simulink model "AnotherOopsies"  (R2020a)
settings: Solver=FixedStepAuto  StartTime=0.0  StopTime=10.0  FixedStep=1e-3  RelTol=1e-3  EnableMultiTasking=on
undefined symbols (not defined in the file or in its folder): A0, A1, D0, D1, D10, D11, D12, D13, D2, D3, D4, D5, D6, D7, D8, D9, PTA0, PTA1, PTA2, PTB2, PTB23, PTB3, PTB9, PTC16, PTC17, PTC2, PTC3, PTC4, PTD0, PTD1, PTD2, PTD3
libraries: frdmk64flib x19, etargetslib x8, dspstat3 x1
settings Model: ExtModeTrigDuration=5  Creator=haque  LastModifiedBy=haque
settings OptimizationCC: EnhancedBackFolding=on  PassReuseOutputArgsAs=Individual arguments  ZeroExternalMemoryAtStartup=off  ZeroInternalMemoryAtStartup=off  MaxStackSize=64  OptimizeBlockOrder=speed  DifferentSizesBufferReuse=on  OptimizationCustomize=off  EfficientTunableParamExpr=on
settings DebuggingCC: ParameterTunabilityLossMsg=error
settings HardwareCC: ProdBitPerPointer=32  ProdBitPerSizeT=32  ProdBitPerPtrDiffT=32  ProdLargestAtomicInteger=Long  ProdLargestAtomicFloat=Double  ProdWordSize=32  ProdHWDeviceType=ARM Compatible->ARM Cortex
settings SFSimCC: MATLABDynamicMemAlloc=off
settings RTWCC: SystemTargetFile=ert.tlc  HardwareBoard=NXP FRDM-K64F  TemplateMakefile=ert_default_tmf  Toolchain=GNU Tools for ARM Embedded Processors
settings CodeAppCC: ForceParamTrailComments=on  IgnoreCustomStorageClasses=off  OperatorAnnotations=on  SimulinkDataObjDesc=on  SFDataObjDesc=on  InsertBlockDesc=on

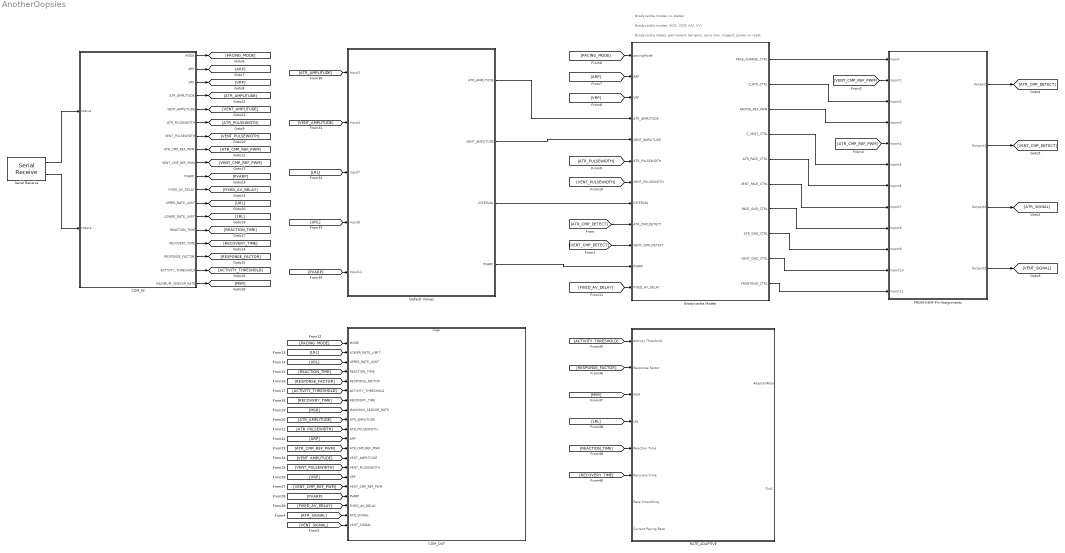
== system AnotherOopsies ==
  note: Bradycardia modes vs. states:
  note: Bradycardia states: permanent, tempory, pace now, magent, power on reset
  note: Bradycardia modes: AOO, VOO, AAI, VVI
  Bradycardia Modes : Stateflow chart  TreatAsAtomicUnit=on
  COM_IN : Stateflow chart  TreatAsAtomicUnit=on
  COM_OUT : Subsystem  TreatAsAtomicUnit=on
  Default Values : Subsystem
  FRDM-K64F Pin Assignments : Subsystem
  RATE_ADAPTIVE : Subsystem
  Serial Receive : frdmk64flib/Serial Receive  SCIModule=0  Baudrate=uint32(9600)  Parity=None  StopBits=1  HardwareFlowControl=None  ByteOrder=LittleEndian  DataType=uint8  DataLength=10  BlockingMode=off  OutputStatus=on  SampleTime=0.1
  wires:
  Bradycardia Modes/1(PACE_CHARGE_CTRL) -> FRDM-K64F Pin Assignments/1(Inport)
  Bradycardia Modes/2(Z_ATR_CTRL) -> FRDM-K64F Pin Assignments/3(Inport2)
  Bradycardia Modes/3(PACING_REF_PWM) -> FRDM-K64F Pin Assignments/4(Inport3)
  Bradycardia Modes/4(Z_VENT_CTRL) -> FRDM-K64F Pin Assignments/6(Inport5)
  Bradycardia Modes/5(ATR_PACE_CTRL) -> FRDM-K64F Pin Assignments/7(Inport6)
  Bradycardia Modes/6(VENT_PACE_CTRL) -> FRDM-K64F Pin Assignments/8(Inport7)
  Bradycardia Modes/7(PACE_GND_CTRL) -> FRDM-K64F Pin Assignments/9(Inport8)
  Bradycardia Modes/8(ATR_GND_CTRL) -> FRDM-K64F Pin Assignments/10(Inport9)
  Bradycardia Modes/9(VENT_GND_CTRL) -> FRDM-K64F Pin Assignments/11(Inport10)
  Bradycardia Modes/10(FRONTEND_CTRL) -> FRDM-K64F Pin Assignments/12(Inport11)
  Default Values/3(INTERVAL) -> Bradycardia Modes/8(INTERVAL)
  Default Values/2(VENT_AMPLITUDE) -> Bradycardia Modes/5(VENT_AMPLITUDE)
  Default Values/1(ATR_AMPLITUDE) -> Bradycardia Modes/4(ATR_AMPLITUDE)
  FRDM-K64F Pin Assignments/1(Outport) -> [ATR_CMP_DETECT]
  FRDM-K64F Pin Assignments/2(Outport1) -> [VENT_CMP_DETECT]
  [ATR_CMP_DETECT] -> Bradycardia Modes/9(ATR_CMP_DETECT)
  [VENT_CMP_DETECT] -> Bradycardia Modes/10(VENT_CMP_DETECT)
  [VENT_CMP_REF_PWM] -> FRDM-K64F Pin Assignments/2(Inport1)
  [ATR_CMP_REF_PWM] -> FRDM-K64F Pin Assignments/5(Inport4)
  Serial Receive/1 -> COM_IN/1(status)
  Serial Receive/2 -> COM_IN/2(rxdata)
  FRDM-K64F Pin Assignments/3(Outport2) -> [ATR_SIGNAL]
  FRDM-K64F Pin Assignments/4(Outport3) -> [VENT_SIGNAL]
  [ATR_SIGNAL] -> COM_OUT/19(ATR_SIGNAL)
  [VENT_SIGNAL] -> COM_OUT/20(VENT_SIGNAL)
  Default Values/4(PVARP) -> Bradycardia Modes/11(PVARP)
  [PACING_MODE] -> Bradycardia Modes/1(pacingMode)
  [ARP] -> Bradycardia Modes/2(ARP)
  [VRP] -> Bradycardia Modes/3(VRP)
  [VENT_PULSEWIDTH] -> Bradycardia Modes/7(VENT_PULSEWIDTH)
  [FIXED_AV_DELAY] -> Bradycardia Modes/12(FIXED_AV_DELAY)
  [ATR_PULSEWIDTH] -> Bradycardia Modes/6(ATR_PULSEWIDTH)
  [PACING_MODE] -> COM_OUT/1(MODE)
  [LRL] -> COM_OUT/2(LOWER_RATE_LIMIT)
  [REACTION_TIME] -> COM_OUT/4(REACTION_TIME)
  [URL] -> COM_OUT/3(UPPER_RATE_LIMIT)
  [MSR] -> COM_OUT/8(MAXIMUM_SENSOR_RATE)
  [RESPONSE_FACTOR] -> COM_OUT/5(RESPONSE_FACTOR)
  [ACTIVITY_THRESHOLD] -> COM_OUT/6(ACTIVITY_THRESHOLD)
  [RECOVERY_TIME] -> COM_OUT/7(RECOVERY_TIME)
  [ATR_AMPLITUDE] -> COM_OUT/9(ATR_AMPLITUDE)
  [ATR_PULSEWIDTH] -> COM_OUT/10(ATR_PULSEWIDTH)
  [ARP] -> COM_OUT/11(ARP)
  [ATR_CMP_REF_PWM] -> COM_OUT/12(ATR_CMP_REF_PWM)
  [VENT_AMPLITUDE] -> COM_OUT/13(VENT_AMPLITUDE)
  [VENT_PULSEWIDTH] -> COM_OUT/14(VENT_PULSEWIDTH)
  [VRP] -> COM_OUT/15(VRP)
  [VENT_CMP_REF_PWM] -> COM_OUT/16(VENT_CMP_REF_PWM)
  [FIXED_AV_DELAY] -> COM_OUT/18(FIXED_AV_DELAY)
  [PVARP] -> COM_OUT/17(PVARP)
  COM_IN/1(MODE) -> [PACING_MODE]
  COM_IN/2(ARP) -> [ARP]
  COM_IN/3(VRP) -> [VRP]
  COM_IN/7(VENT_PULSEWIDTH) -> [VENT_PULSEWIDTH]
  COM_IN/6(ATR_PULSEWIDTH) -> [ATR_PULSEWIDTH]
  COM_IN/8(ATR_CMP_REF_PWM) -> [ATR_CMP_REF_PWM]
  COM_IN/9(VENT_CMP_REF_PWM) -> [VENT_CMP_REF_PWM]
  COM_IN/11(FIXED_AV_DELAY) -> [FIXED_AV_DELAY]
  COM_IN/16(RESPONSE_FACTOR) -> [RESPONSE_FACTOR]
  COM_IN/18(MAXIMUM_SENSOR_RATE) -> [MSR]
  COM_IN/17(ACTIVITY_THRESHOLD) -> [ACTIVITY_THRESHOLD]
  COM_IN/15(RECOVERY_TIME) -> [RECOVERY_TIME]
  COM_IN/14(REACTION_TIME) -> [REACTION_TIME]
  COM_IN/12(UPPER_RATE_LIMIT) -> [URL]
  COM_IN/13(LOWER_RATE_LIMIT) -> [LRL]
  COM_IN/4(ATR_AMPLITUDE) -> [ATR_AMPLITUDE]
  COM_IN/5(VENT_AMPLITUDE) -> [VENT_AMPLITUDE]
  COM_IN/10(PVARP) -> [PVARP]
  [ATR_AMPLITUDE] -> Default Values/1(Input3)
  [VENT_AMPLITUDE] -> Default Values/2(Input4)
  [LRL] -> Default Values/3(Input7)
  [URL] -> Default Values/4(Input8)
  [PVARP] -> Default Values/5(Input11)
  [ACTIVITY_THRESHOLD] -> RATE_ADAPTIVE/1(Activity Threshold)
  [RESPONSE_FACTOR] -> RATE_ADAPTIVE/2(Response Factor)
  [MSR] -> RATE_ADAPTIVE/3(MSR)
  [LRL] -> RATE_ADAPTIVE/4(LRL)
  [REACTION_TIME] -> RATE_ADAPTIVE/5(Reaction Time)
  [RECOVERY_TIME] -> RATE_ADAPTIVE/6(Recovery Time)

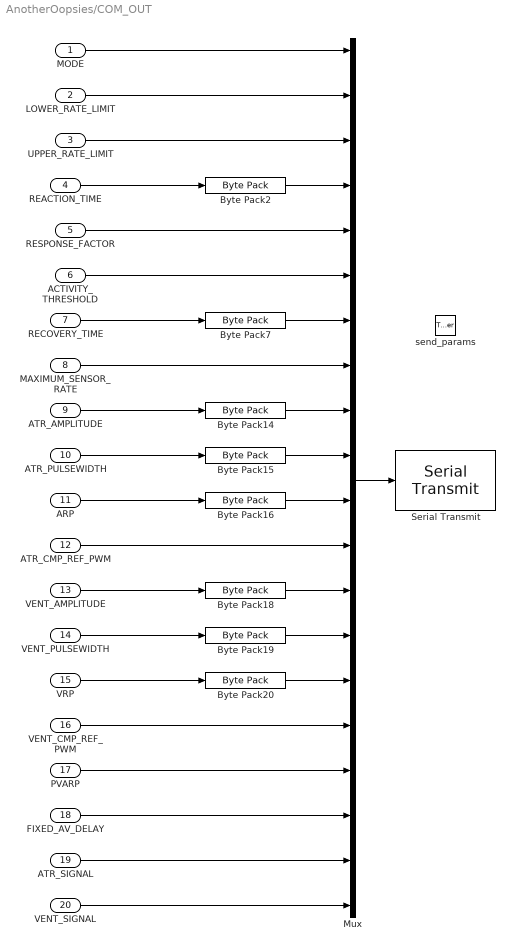
== system AnotherOopsies/COM_OUT ==
  MODE : Inport
  LOWER_RATE_LIMIT : Inport  Port=2
  UPPER_RATE_LIMIT : Inport  Port=3
  REACTION_TIME : Inport  Port=4
  RESPONSE_FACTOR : Inport  Port=5
  ACTIVITY_THRESHOLD : Inport  Port=6
  RECOVERY_TIME : Inport  Port=7
  MAXIMUM_SENSOR_RATE : Inport  Port=8
  ATR_AMPLITUDE : Inport  Port=9
  ATR_PULSEWIDTH : Inport  Port=10
  ARP : Inport  Port=11
  ATR_CMP_REF_PWM : Inport  Port=12
  VENT_AMPLITUDE : Inport  Port=13
  VENT_PULSEWIDTH : Inport  Port=14
  VRP : Inport  Port=15
  VENT_CMP_REF_PWM : Inport  Port=16
  PVARP : Inport  Port=17
  FIXED_AV_DELAY : Inport  Port=18
  ATR_SIGNAL : Inport  Port=19
  VENT_SIGNAL : Inport  Port=20
  send_params : TriggerPort  TriggerType=function-call  IsSimulinkFunction=on  FunctionName=send_params  VariantControl=Variant
  Byte Pack14 : etargetslib/Byte Pack  datatypes={'single'}  byteAlign=1
  Byte Pack{2,7,15..16,19..20} (6 alike) : etargetslib/Byte Pack  datatypes={'uint16'}  byteAlign=1
  Byte Pack18 : etargetslib/Byte Pack  datatypes={'single'}  byteAlign=1
  Mux : Mux  Inputs=20
  Serial Transmit : frdmk64flib/Serial Transmit  SCIModule=0  Baudrate=uint32(9600)  Parity=None  StopBits=1  HardwareFlowControl=None  ByteOrder=LittleEndian  BlockingMode=on  OutputStatus=off
  wires:
  LOWER_RATE_LIMIT/1 -> Mux/2
  RECOVERY_TIME/1 -> Byte Pack7/1
  REACTION_TIME/1 -> Byte Pack2/1
  ATR_AMPLITUDE/1 -> Byte Pack14/1
  ACTIVITY_THRESHOLD/1 -> Mux/6
  Byte Pack2/1 -> Mux/4
  MAXIMUM_SENSOR_RATE/1 -> Mux/8
  VENT_CMP_REF_PWM/1 -> Mux/16
  UPPER_RATE_LIMIT/1 -> Mux/3
  ATR_PULSEWIDTH/1 -> Byte Pack15/1
  Byte Pack7/1 -> Mux/7
  RESPONSE_FACTOR/1 -> Mux/5
  ATR_CMP_REF_PWM/1 -> Mux/12
  VRP/1 -> Byte Pack20/1
  MODE/1 -> Mux/1
  VENT_PULSEWIDTH/1 -> Byte Pack19/1
  VENT_AMPLITUDE/1 -> Byte Pack18/1
  Mux/1 -> Serial Transmit/1
  Byte Pack20/1 -> Mux/15
  Byte Pack18/1 -> Mux/13
  PVARP/1 -> Mux/17
  Byte Pack15/1 -> Mux/10
  Byte Pack14/1 -> Mux/9
  ARP/1 -> Byte Pack16/1
  Byte Pack19/1 -> Mux/14
  FIXED_AV_DELAY/1 -> Mux/18
  Byte Pack16/1 -> Mux/11
  ATR_SIGNAL/1 -> Mux/19
  VENT_SIGNAL/1 -> Mux/20

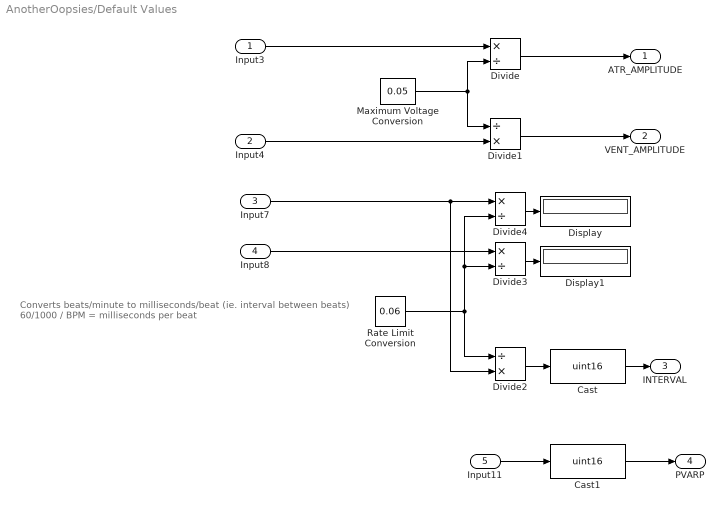
== system AnotherOopsies/Default Values ==
  note: Converts beats/minute to milliseconds/beat (ie. interval between beats)
      | 60/1000 / BPM = milliseconds per beat
  Input3 : Inport
  Input4 : Inport  Port=2
  Input7 : Inport  Port=3
  Input8 : Inport  Port=4
  Input11 : Inport  Port=5
  Cast : DataTypeConversion  OutDataTypeStr=uint16  LockScale=on
  Cast1 : DataTypeConversion  OutDataTypeStr=uint16  LockScale=on
  Display : Display
  Display1 : Display
  Divide : Product  Inputs=*/
  Divide1 : Product  Inputs=/*
  Divide2 : Product  Inputs=/*
  Divide3 : Product  Inputs=*/
  Divide4 : Product  Inputs=*/
  Maximum Voltage Conversion : Constant  Value=0.05
  Rate Limit Conversion : Constant  Value=0.06
  ATR_AMPLITUDE : Outport
  VENT_AMPLITUDE : Outport  Port=2
  INTERVAL : Outport  Port=3
  PVARP : Outport  Port=4
  wires:
  Input3/1 -> Divide/1
  Maximum Voltage Conversion/1 -> Divide1/1, Divide/2
  Divide/1 -> ATR_AMPLITUDE/1
  Divide1/1 -> VENT_AMPLITUDE/1
  Input4/1 -> Divide1/2
  Input8/1 -> Divide3/1
  Input7/1 -> Divide2/2, Divide4/1
  Divide4/1 -> Display/1
  Divide3/1 -> Display1/1
  Rate Limit Conversion/1 -> Divide3/2, Divide4/2, Divide2/1
  Divide2/1 -> Cast/1
  Cast/1 -> INTERVAL/1
  Input11/1 -> Cast1/1
  Cast1/1 -> PVARP/1

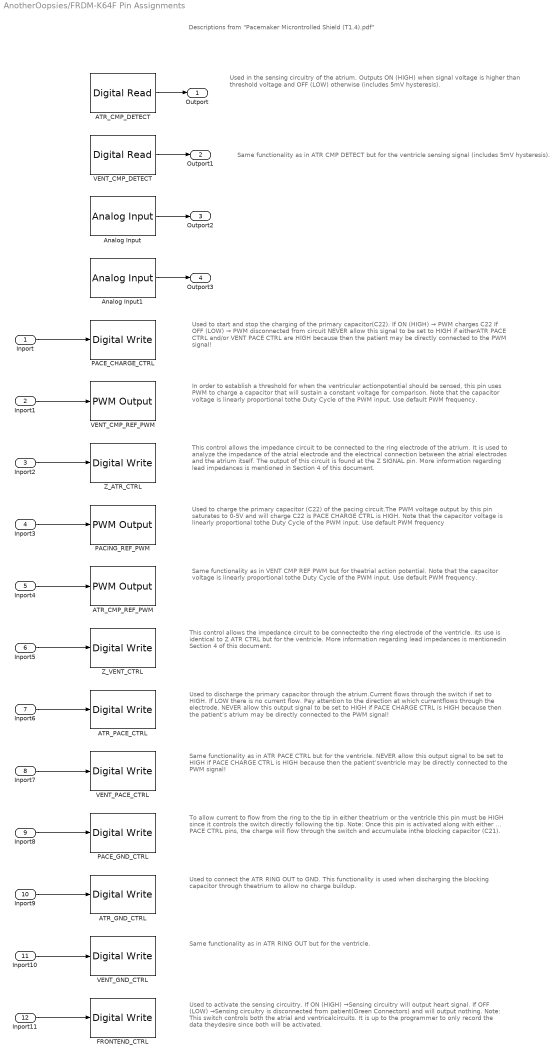
== system AnotherOopsies/FRDM-K64F Pin Assignments ==
  note: Used to activate the sensing circuitry.
      | If ON (HIGH) →Sensing circuitry will output heart signal.
      | If OFF (LOW) →Sensing circuitry is disconnected from patient(Green Connectors) and will output nothing.
      |
      | Note: This switch controls both the atrial and ventricalcircuits. It is up to the programmer to only record the data theydesire since both will be activated.
  note: Same functionality as in ATR RING OUT but for the ventricle.
  note: This control allows the impedance circuit to be connectedto the ring electrode of the ventricle. Its use is identical to Z ATR CTRL but for the ventricle.
      | More information regarding lead impedances is mentionedin Section 4 of this document.
  note: Same functionality as in VENT CMP REF PWM but for theatrial action potential.
      | Note that the capacitor voltage is linearly proportional tothe Duty Cycle of the PWM input. Use default PWM frequency.
  note: This control allows the impedance circuit to be connected to the ring electrode of the atrium.
      | It is used to analyze the impedance of the atrial electrode and the electrical connection between the atrial electrodes and the atrium itself.
      | The output of this circuit is found at the Z SIGNAL pin. More information regarding lead impedances is mentioned in Section 4 of this document.
  note: Descriptions from "Pacemaker Microntrolled Shield (T1.4).pdf"
  note: In order to establish a threshold for when the ventricular actionpotential should be sensed, this pin uses PWM to charge a capacitor that will sustain a constant voltage for comparison.
      | Note that the capacitor voltage is linearly proportional tothe Duty Cycle of the PWM input. Use default PWM frequency.
  note: Used to charge the primary capacitor (C22) of the pacing circuit.The PWM voltage output by this pin saturates to 0-5V and will charge C22 is PACE CHARGE CTRL is HIGH.
      | Note that the capacitor voltage is linearly proportional tothe Duty Cycle of the PWM input. Use default PWM frequency
  note: Used to start and stop the charging of the primary capacitor(C22).
      | If ON (HIGH) → PWM charges C22
      | If OFF (LOW) → PWM disconnected from circuit
      | NEVER allow this signal to be set to HIGH if eitherATR PACE CTRL and/or VENT PACE CTRL are HIGH because then the patient may be directly connected to the PWM signal!
  note: To allow current to flow from the ring to the tip in either theatrium or the ventricle this pin must be HIGH since it controls the switch directly following the tip.
      | Note: Once this pin is activated along with either ... PACE CTRL pins, the charge will flow through the switch and accumulate inthe blocking capacitor (C21).
  note: Same functionality as in ATR CMP DETECT but for the ventricle sensing signal (includes 5mV hysteresis).
  note: Same functionality as in ATR PACE CTRL but for the ventricle.
      | NEVER allow this output signal to be set to HIGH if PACE CHARGE CTRL is HIGH because then the patient’sventricle may be directly connected to the PWM signal!
  note: Used in the sensing circuitry of the atrium. Outputs ON (HIGH) when signal voltage is higher than threshold voltage and OFF (LOW) otherwise (includes 5mV hysteresis).
  note: Used to discharge the primary capacitor through the atrium.Current flows through the switch if set to HIGH. If LOW there is no current flow. Pay attention to the direction at which currentflows through the electrode.
      | NEVER allow this output signal to be set to HIGH if PACE CHARGE CTRL is HIGH because then the patient’s atrium may be directly connected to the PWM signal!
  note: Used to connect the ATR RING OUT to GND. This functionality is used when discharging the blocking capacitor through theatrium to allow no charge buildup.
  Inport : Inport
  Inport1 : Inport  Port=2
  Inport2 : Inport  Port=3
  Inport3 : Inport  Port=4
  Inport4 : Inport  Port=5
  Inport5 : Inport  Port=6
  Inport6 : Inport  Port=7
  Inport7 : Inport  Port=8
  Inport8 : Inport  Port=9
  Inport9 : Inport  Port=10
  Inport10 : Inport  Port=11
  Inport11 : Inport  Port=12
  ATR_CMP_DETECT : frdmk64flib/Digital Read  Whichpin=PTC16 (D0)  SampleTime=-1
  ATR_CMP_REF_PWM : frdmk64flib/PWM Output  Whichpin=PTC2 (D6)  InitialFrequency=2000  InitialDutyCycle=30
  ATR_GND_CTRL : frdmk64flib/Digital Write  Whichpin=PTD2 (D11)
  ATR_PACE_CTRL : frdmk64flib/Digital Write  Whichpin=PTA0 (D8)
  Analog Input : frdmk64flib/Analog Input  Whichpin=PTB2 (A0)  SampleTime=-1
  Analog Input1 : frdmk64flib/Analog Input  Whichpin=PTB3 (A1)  SampleTime=-1
  FRONTEND_CTRL : frdmk64flib/Digital Write  Whichpin=PTD1 (D13)
  PACE_CHARGE_CTRL : frdmk64flib/Digital Write  Whichpin=PTB9 (D2)
  PACE_GND_CTRL : frdmk64flib/Digital Write  Whichpin=PTD0 (D10)
  PACING_REF_PWM : frdmk64flib/PWM Output  Whichpin=PTA2 (D5)  InitialFrequency=2000  InitialDutyCycle=30
  VENT_CMP_DETECT : frdmk64flib/Digital Read  Whichpin=PTC17 (D1)  SampleTime=-1
  VENT_CMP_REF_PWM : frdmk64flib/PWM Output  Whichpin=PTA1 (D3)  InitialFrequency=2000  InitialDutyCycle=30
  VENT_GND_CTRL : frdmk64flib/Digital Write  Whichpin=PTD3 (D12)
  VENT_PACE_CTRL : frdmk64flib/Digital Write  Whichpin=PTC4 (D9)
  Z_ATR_CTRL : frdmk64flib/Digital Write  Whichpin=PTB23 (D4)
  Z_VENT_CTRL : frdmk64flib/Digital Write  Whichpin=PTC3 (D7)
  Outport : Outport
  Outport1 : Outport  Port=2
  Outport2 : Outport  Port=3
  Outport3 : Outport  Port=4
  wires:
  Inport10/1 -> VENT_GND_CTRL/1
  Inport9/1 -> ATR_GND_CTRL/1
  Inport1/1 -> VENT_CMP_REF_PWM/1
  Inport7/1 -> VENT_PACE_CTRL/1
  Inport2/1 -> Z_ATR_CTRL/1
  Inport8/1 -> PACE_GND_CTRL/1
  Inport3/1 -> PACING_REF_PWM/1
  Inport4/1 -> ATR_CMP_REF_PWM/1
  VENT_CMP_DETECT/1 -> Outport1/1
  Inport5/1 -> Z_VENT_CTRL/1
  Inport11/1 -> FRONTEND_CTRL/1
  Inport6/1 -> ATR_PACE_CTRL/1
  ATR_CMP_DETECT/1 -> Outport/1
  Inport/1 -> PACE_CHARGE_CTRL/1
  Analog Input/1 -> Outport2/1
  Analog Input1/1 -> Outport3/1

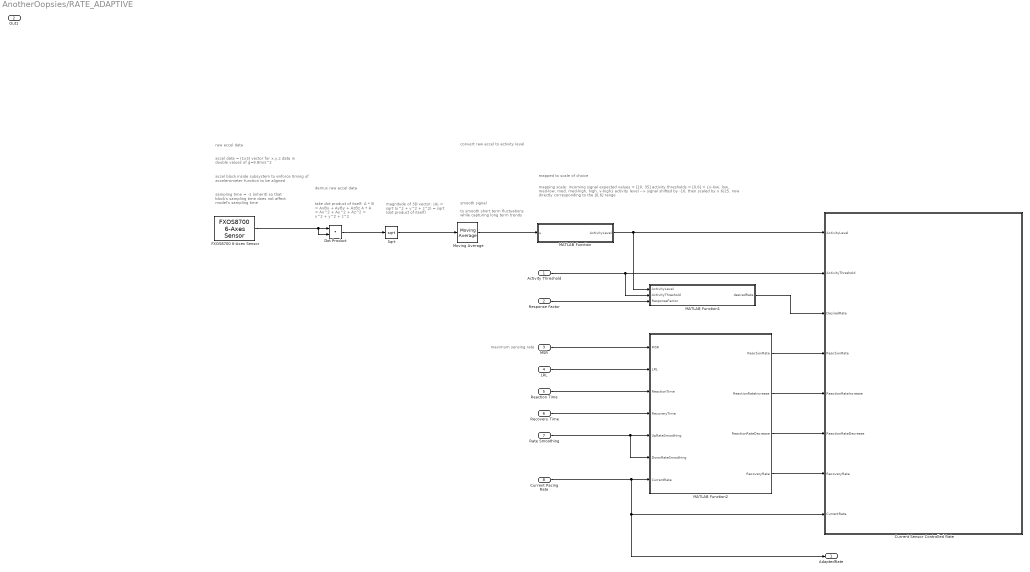
== system AnotherOopsies/RATE_ADAPTIVE ==
  note: demux raw accel data
  note: accel block inside subsystem to enforce timing
      |  of accelerometer function to be aligned
  note: to smooth short term fluctuations
      | while capturing long term trends
  note: smooth signal
  note: sampling time = -1 (inherit)
      |
      | so that block's sampling time does
      | not affect model's sampling time
  note: raw accel data
  note: mapped to scale of choice
  note: maximum sensing rate
  note: convert raw accel to activity level
  note: mapping scale:
      |
      | incoming signal expected values = [10, 35]
      | activity thresholds = [0,6]
      | 				 = {v-low, low, med-low, med, med-high, high, v-high}
      |
      | activity level --> signal shifted by -10, then scaled by x 6/25, now directly corresponding to the [0,6] range
  note: take dot product of itself:
      | A * B = AxBx + AyBy + AzBz
      | A * A = Ax^2 + Ay^2 + Az^2
      |          = x^2 + y^2 + z^2
  note: magnitude of 3D vector:
      | |A| = sqrt (x^2 + y^2 + z^2)
      |      = sqrt (dot product of itself)
  note: accel data = [1x3] vector for x,y,z data
      | in double values of g=9.8m/s^2
  Activity Threshold : Inport
  Response Factor : Inport  Port=2
  MSR : Inport  Port=3
  LRL : Inport  Port=4
  Reaction Time : Inport  Port=5
  Recovery Time : Inport  Port=6
  Rate Smoothing : Inport  Port=7
  Current Pacing Rate : Inport  Port=8
  Current Sensor Controlled Rate : Stateflow chart  TreatAsAtomicUnit=on
  Dot Product : DotProduct  InputSameDT=on  OutDataTypeStr=Inherit: Inherit via internal rule
  FXOS8700 6-Axes Sensor : frdmk64flib/FXOS8700 6-Axes Sensor  Activesensor=Accelerometer only  ODR=800Hz  HybridODR=400Hz  Accelfullrange=-4g to +4g  SampleTime=-1
  MATLAB Function : MATLAB Function  TreatAsAtomicUnit=on
  MATLAB Function1 : MATLAB Function  TreatAsAtomicUnit=on
  MATLAB Function2 : MATLAB Function  TreatAsAtomicUnit=on
  Moving Average : dspstat3/Moving Average  Method=Sliding window  ForgettingFactorPort=off  SpecifyWindowLength=on  WindowLength=4  ForgettingFactor=0.9  SimulateUsing=Code generation
  Sqrt : Sqrt  SaturateOnIntegerOverflow=on
  AdaptedRate : Outport
  Out1 : Outport  Port=2
  wires:
  MSR/1 -> MATLAB Function2/1(MSR)
  FXOS8700 6-Axes Sensor/1 -> Dot Product/2, Dot Product/1
  Response Factor/1 -> MATLAB Function1/3(ResponseFactor)
  Moving Average/1 -> MATLAB Function/1(u)
  Dot Product/1 -> Sqrt/1
  MATLAB Function/1(ActivityLevel) -> MATLAB Function1/1(ActivityLevel), Current Sensor Controlled Rate/1(ActivityLevel)
  Sqrt/1 -> Moving Average/1
  MATLAB Function2/4(RecoveryRate) -> Current Sensor Controlled Rate/7(RecoveryRate)
  Recovery Time/1 -> MATLAB Function2/4(RecoveryTime)
  MATLAB Function2/1(ReactionRate) -> Current Sensor Controlled Rate/4(ReactionRate)
  Reaction Time/1 -> MATLAB Function2/3(ReactionTime)
  Rate Smoothing/1 -> MATLAB Function2/6(DownRateSmoothing), MATLAB Function2/5(UpRateSmoothing)
  MATLAB Function2/2(ReactionRateIncrease) -> Current Sensor Controlled Rate/5(ReactionRateIncrease)
  MATLAB Function2/3(ReactionRateDecrease) -> Current Sensor Controlled Rate/6(ReactionRateDecrease)
  Activity Threshold/1 -> MATLAB Function1/2(ActivityThreshold), Current Sensor Controlled Rate/2(ActivityThreshold)
  LRL/1 -> MATLAB Function2/2(LRL)
  MATLAB Function1/1(desiredRate) -> Current Sensor Controlled Rate/3(DesiredRate)
  Current Pacing Rate/1 -> Current Sensor Controlled Rate/8(CurrentRate), AdaptedRate/1, MATLAB Function2/7(CurrentRate)

== stateflow chart AnotherOopsies/Bradycardia Modes ==
  state AOOR
    state Wait_Charging
      entry:
      %charging C22 (pg.11)
      ATR_PACE_CTRL = 0
      VENT_PACE_CTRL = 0
      PACING_REF_PWM = ATR_AMPLITUDE;  % sets amplitude (duty cycle)
      PACE_CHARGE_CTRL = 1
      %release C21
      PACE_GND_CTRL = 1
      VENT_GND_CTRL = 0
      Z_ATR_CTRL = 0
      Z_VENT_CTRL = 0
      ATR_PACE_CTRL = 0
      ATR_GND_CTRL = 1
      VENT_GND_CTRL = 0
    state Pace_Discharging
      entry:
      %release C22 to charge C21
      PACE_CHARGE_CTRL = 0
      PACE_GND_CTRL = 1
      VENT_PACE_CTRL = 0
      VENT_GND_CTRL = 0
      Z_VENT_CTRL = 0
      Z_ATR_CTRL = 0
      ATR_GND_CTRL = 0
      ATR_PACE_CTRL = 1
    (default) -> AOOR.Wait_Charging
    AOOR.Wait_Charging -> AOOR.Pace_Discharging : [after(INTERVAL, msec)]
    AOOR.Pace_Discharging -> AOOR.Wait_Charging : [after(ATR_PULSEWIDTH,msec)]
  state AOO
    state Wait_Charging
      entry:
      %charging C22 (pg.11)
      ATR_PACE_CTRL = 0
      VENT_PACE_CTRL = 0
      PACING_REF_PWM = ATR_AMPLITUDE;  % sets amplitude (duty cycle)
      PACE_CHARGE_CTRL = 1
      %release C21
      PACE_GND_CTRL = 1
      VENT_GND_CTRL = 0
      Z_ATR_CTRL = 0
      Z_VENT_CTRL = 0
      ATR_PACE_CTRL = 0
      ATR_GND_CTRL = 1
      VENT_GND_CTRL = 0
    state Pace_Discharging
      entry:
      %release C22 to charge C21
      PACE_CHARGE_CTRL = 0
      PACE_GND_CTRL = 1
      VENT_PACE_CTRL = 0
      VENT_GND_CTRL = 0
      Z_VENT_CTRL = 0
      Z_ATR_CTRL = 0
      ATR_GND_CTRL = 0
      ATR_PACE_CTRL = 1
    (default) -> AOO.Wait_Charging
    AOO.Wait_Charging -> AOO.Pace_Discharging : [after(INTERVAL, msec)]
    AOO.Pace_Discharging -> AOO.Wait_Charging : [after(ATR_PULSEWIDTH,msec)]
  state PacingModes
    %chooses a pacing mode
    %{
    defined pacingModes:
    AOO = 0
    VOO = 1
    AAI = 2
    VVI = 3
    %}
  state VOOR
    state Wait_Charging
      entry:
      ATR_PACE_CTRL = 0;
      VENT_PACE_CTRL = 0;
      PACE_CHARGE_CTRL = 1;
      PACING_REF_PWM = VENT_AMPLITUDE;  % sets amplitude (duty cycle)
      PACE_GND_CTRL = 1;
      VENT_GND_CTRL = 1;
      ATR_GND_CTRL = 0;
      Z_ATR_CTRL = 0;
      Z_VENT_CTRL = 0;
    state Pace_Discharging
      entry:
      PACE_GND_CTRL = 1
      VENT_PACE_CTRL = 1
      VENT_GND_CTRL = 0
      Z_VENT_CTRL = 0
      Z_ATR_CTRL = 0
      ATR_GND_CTRL = 0
      ATR_PACE_CTRL = 0
      PACE_CHARGE_CTRL = 0;
    (default) -> VOOR.Wait_Charging
    VOOR.Wait_Charging -> VOOR.Pace_Discharging : [after(INTERVAL, msec)]
    VOOR.Pace_Discharging -> VOOR.Wait_Charging : [after(VENT_PULSEWIDTH, msec)]
  state VOO
    state Wait_Charging
      entry:
      ATR_PACE_CTRL = 0;
      VENT_PACE_CTRL = 0;
      PACE_CHARGE_CTRL = 1;
      PACING_REF_PWM = VENT_AMPLITUDE;  % sets amplitude (duty cycle)
      PACE_GND_CTRL = 1;
      VENT_GND_CTRL = 1;
      ATR_GND_CTRL = 0;
      Z_ATR_CTRL = 0;
      Z_VENT_CTRL = 0;
    state Pace_Discharging
      entry:
      PACE_GND_CTRL = 1
      VENT_PACE_CTRL = 1
      VENT_GND_CTRL = 0
      Z_VENT_CTRL = 0
      Z_ATR_CTRL = 0
      ATR_GND_CTRL = 0
      ATR_PACE_CTRL = 0
      PACE_CHARGE_CTRL = 0;
    (default) -> VOO.Wait_Charging
    VOO.Wait_Charging -> VOO.Pace_Discharging : [after(INTERVAL, msec)]
    VOO.Pace_Discharging -> VOO.Wait_Charging : [after(VENT_PULSEWIDTH, msec)]
  state AAIR
    state Charging_C22_Discharging_C21
      entry:
      % Turn on sensing:
      FRONTEND_CTRL = 1
      %Charging C22 Capacitor:
      ATR_PACE_CTRL = 0
      VENT_PACE_CTRL = 0
      PACING_REF_PWM = ATR_AMPLITUDE
      PACE_CHARGE_CTRL = 1
      %
      % Discharging C21 Capacitor
      PACE_GND_CTRL = 1
      VENT_PACE_CTRL = 0
      Z_ATR_CTRL = 0
      Z_VENT_CTRL = 0
      ATR_PACE_CTRL = 0
      VENT_GND_CTRL = 0
      ATR_GND_CTRL = 1
    state Sensing_Heartbeat
      %after ARP, check sense
    state Discharging_C22_Charging_C21
      %AV Pace
      PACE_CHARGE_CTRL = 0
      PACE_GND_CTRL = 1
      ATR_PACE_CTRL = 0
      ATR_GND_CTRL = 0
      Z_ATR_CTRL = 0
      Z_VENT_CTRL = 0
      VENT_GND_CTRL = 0
      ATR_PACE_CTRL = 1
    (default) -> AAIR.Charging_C22_Discharging_C21
    AAIR.Sensing_Heartbeat -> AAIR.Charging_C22_Discharging_C21 [order 2] : [ATR_CMP_DETECT == 1]
    AAIR.Charging_C22_Discharging_C21 -> AAIR.Sensing_Heartbeat : [after(ARP, msec)]
    AAIR.Sensing_Heartbeat -> AAIR.Discharging_C22_Charging_C21 [order 1] : [after(INTERVAL - ARP, msec)]
    AAIR.Discharging_C22_Charging_C21 -> AAIR.Charging_C22_Discharging_C21 : [after(ATR_PULSEWIDTH, msec)]
  state AAI
    state Charging_C22_Discharging_C21
      entry:
      % Turn on sensing:
      FRONTEND_CTRL = 1
      %Charging C22 Capacitor:
      ATR_PACE_CTRL = 0
      VENT_PACE_CTRL = 0
      PACING_REF_PWM = ATR_AMPLITUDE
      PACE_CHARGE_CTRL = 1
      %
      % Discharging C21 Capacitor
      PACE_GND_CTRL = 1
      VENT_PACE_CTRL = 0
      Z_ATR_CTRL = 0
      Z_VENT_CTRL = 0
      ATR_PACE_CTRL = 0
      VENT_GND_CTRL = 0
      ATR_GND_CTRL = 1
    state Sensing_Heartbeat
      %after ARP, check sense
    state Discharging_C22_Charging_C21
      %AV Pace
      PACE_CHARGE_CTRL = 0
      PACE_GND_CTRL = 1
      ATR_PACE_CTRL = 0
      ATR_GND_CTRL = 0
      Z_ATR_CTRL = 0
      Z_VENT_CTRL = 0
      VENT_GND_CTRL = 0
      ATR_PACE_CTRL = 1
    (default) -> AAI.Charging_C22_Discharging_C21
    AAI.Sensing_Heartbeat -> AAI.Charging_C22_Discharging_C21 [order 2] : [ATR_CMP_DETECT == 1]
    AAI.Charging_C22_Discharging_C21 -> AAI.Sensing_Heartbeat : [after(ARP, msec)]
    AAI.Sensing_Heartbeat -> AAI.Discharging_C22_Charging_C21 [order 1] : [after(INTERVAL - ARP, msec)]
    AAI.Discharging_C22_Charging_C21 -> AAI.Charging_C22_Discharging_C21 : [after(ATR_PULSEWIDTH, msec)]
  state VVIR
    state Charging
      entry:
      % Sensing on:
      FRONTEND_CTRL = 1
      % charging C22 capacitor:
      ATR_PACE_CTRL=0
      VENT_PACE_CTRL=0
      PACING_REF_PWM=VENT_AMPLITUDE
      PACE_CHARGE_CTRL=1
      %
      % Release C21 capacitor charge into ventricle gnd
      PACE_GND_CTRL=1
      VENT_PACE_CTRL=0
      Z_ATR_CTRL=0
      Z_VENT_CTRL=0
      ATR_PACE_CTRL=0
      ATR_GND_CTRL=0
      VENT_GND_CTRL=1
      %
      %
      %{
      Purpose: To charge the main pacing capacitor (C22) to a specific voltage, which determines the pacing pulse amplitude.
      What it does: It connects a PWM signal to the capacitor, allowing it to charge up. It also prepares the output circuit for a ventricular pace by connecting the ventricle tip to ground.
      Key Variables/Pins:
      PACE_CHARGE_CTRL = HIGH: This is the main switch that allows the PWM signal to charge capacitor C22.
      PACING_REF_PWM = VENT_AMPLITUDE: This PWM signal's duty cycle determines the final voltage on the capacitor, and thus the strength (amplitude) of the pace.
      VENT_GND_CTRL = HIGH: Prepares the circuit by connecting the ventricle tip to ground, creating a path for the future pacing current.
      FRONTEND_CTRL = HIGH: Turns on the sensing circuitry so the pacemaker can listen for natural heartbeats even while charging.
      %}
    state Transitioning
      % after ventricle refractory period, check sense
    state Discharging
      entry:
      % Release C22 capacitor charge to charge C21 capacitor
      PACE_CHARGE_CTRL=0
      PACE_GND_CTRL=1
      ATR_PACE_CTRL=0
      ATR_GND_CTRL=0
      Z_VENT_CTRL = 0
      Z_ATR_CTRL = 0
      VENT_GND_CTRL = 0
      VENT_PACE_CTRL = 1
      %
      %
      %{
      - To release the energy from capacitor C22 through the heart creating the pacing pulse.
      - It disconnects the charging circuit and connects the charged capacitor (C22) directly to the ventricle ring electrode.
      - The current flows through the heart to the tip (which is grounded), causing the ventricle to contract.
      %}
    (default) -> VVIR.Charging
    VVIR.Transitioning -> VVIR.Charging [order 2] : [VENT_CMP_DETECT == 1]
    VVIR.Discharging -> VVIR.Charging : [after(VENT_PULSEWIDTH,msec)]
    VVIR.Charging -> VVIR.Transitioning : [after(VRP,msec)]
    VVIR.Transitioning -> VVIR.Discharging [order 1] : [after(INTERVAL-VRP,msec)]
  state VVI
    state Charging
      entry:
      % Sensing on:
      FRONTEND_CTRL = 1
      % charging C22 capacitor:
      ATR_PACE_CTRL=0
      VENT_PACE_CTRL=0
      PACING_REF_PWM=VENT_AMPLITUDE
      PACE_CHARGE_CTRL=1
      %
      % Release C21 capacitor charge into ventricle gnd
      PACE_GND_CTRL=1
      VENT_PACE_CTRL=0
      Z_ATR_CTRL=0
      Z_VENT_CTRL=0
      ATR_PACE_CTRL=0
      ATR_GND_CTRL=0
      VENT_GND_CTRL=1
      %
      %
      %{
      Purpose: To charge the main pacing capacitor (C22) to a specific voltage, which determines the pacing pulse amplitude.
      What it does: It connects a PWM signal to the capacitor, allowing it to charge up. It also prepares the output circuit for a ventricular pace by connecting the ventricle tip to ground.
      Key Variables/Pins:
      PACE_CHARGE_CTRL = HIGH: This is the main switch that allows the PWM signal to charge capacitor C22.
      PACING_REF_PWM = VENT_AMPLITUDE: This PWM signal's duty cycle determines the final voltage on the capacitor, and thus the strength (amplitude) of the pace.
      VENT_GND_CTRL = HIGH: Prepares the circuit by connecting the ventricle tip to ground, creating a path for the future pacing current.
      FRONTEND_CTRL = HIGH: Turns on the sensing circuitry so the pacemaker can listen for natural heartbeats even while charging.
      %}
    state Transitioning
      % after ventricle refractory period, check sense
    state Discharging
      entry:
      % Release C22 capacitor charge to charge C21 capacitor
      PACE_CHARGE_CTRL=0
      PACE_GND_CTRL=1
      ATR_PACE_CTRL=0
      ATR_GND_CTRL=0
      Z_VENT_CTRL = 0
      Z_ATR_CTRL = 0
      VENT_GND_CTRL = 0
      VENT_PACE_CTRL = 1
      %
      %
      %{
      - To release the energy from capacitor C22 through the heart creating the pacing pulse.
      - It disconnects the charging circuit and connects the charged capacitor (C22) directly to the ventricle ring electrode.
      - The current flows through the heart to the tip (which is grounded), causing the ventricle to contract.
      %}
    (default) -> VVI.Charging
    VVI.Transitioning -> VVI.Charging [order 2] : [VENT_CMP_DETECT == 1]
    VVI.Discharging -> VVI.Charging : [after(VENT_PULSEWIDTH,msec)]
    VVI.Charging -> VVI.Transitioning : [after(VRP,msec)]
    VVI.Transitioning -> VVI.Discharging [order 1] : [after(INTERVAL-VRP,msec)]
  (default) -> PacingModes
  PacingModes -> AOO [order 7] : [pacingMode==0]
  PacingModes -> AOOR [order 8] : [pacingMode==4]
  PacingModes -> VOOR [order 5] : [pacingMode==5]
  PacingModes -> VOO [order 1] : [pacingMode==1]
  PacingModes -> AAIR [order 4] : [pacingMode==6]
  PacingModes -> AAI [order 2] : [pacingMode==2]
  PacingModes -> VVI [order 6] : [pacingMode==3]
  PacingModes -> VVIR [order 3] : [pacingMode==7]
  data: PACE_CHARGE_CTRL output; Z_ATR_CTRL output; PACING_REF_PWM output; Z_VENT_CTRL output; pacingMode input; ARP input; VRP input; ATR_AMPLITUDE input; VENT_AMPLITUDE input; ATR_PULSEWIDTH input; VENT_PULSEWIDTH input; INTERVAL input; ATR_CMP_DETECT input; VENT_CMP_DETECT input; ATR_PACE_CTRL output; VENT_PACE_CTRL output; PACE_GND_CTRL output; ATR_GND_CTRL output; VENT_GND_CTRL output; FRONTEND_CTRL output; HIGH local =1; FIRST_CYCLE local; PVARP input; FIXED_AV_DELAY input

== stateflow chart AnotherOopsies/RATE_ADAPTIVE/Current Sensor Controlled Rate ==
  state RateAdaptiveIncrease
    entry:
    CurrentRate = CurrentRate + ReactionRateIncrease;
  state RateAdaptiveDecrease
    entry:
    CurrentRate = CurrentRate - ReactionRateDecrease;
  state RateAdaptiveTransition
    % will only remain in this state when ActivityLevel = ActivityThreshold
  state DisableRateAdaptive
    entry:
    CurrentRate = CurrentRate - RecoveryRate;
  RateAdaptiveDecrease -> RateAdaptiveDecrease [order 2] : after(1,msec)
  RateAdaptiveIncrease -> RateAdaptiveIncrease [order 2] : after(1,msec)
  (junction 35) -> RateAdaptiveIncrease [order 2] : [CurrentRate < DesiredRate]
  (junction 35) -> RateAdaptiveDecrease [order 3] : [CurrentRate > DesiredRate]
  RateAdaptiveIncrease -> (junction 35) [order 1] : [(CurrentRate >= DesiredRate) || (ActivityLevel < ActivityThreshold)]
  RateAdaptiveDecrease -> (junction 35) [order 1] : [(CurrentRate <= DesiredRate) || (ActivityLevel < ActivityThreshold)]
  (junction 35) -> RateAdaptiveTransition [order 1] : [ActivityLevel <= ActivityThreshold]
  RateAdaptiveTransition -> (junction 35) [order 1] : [ActivityLevel > ActivityThreshold]
  (default) -> RateAdaptiveTransition
  RateAdaptiveTransition -> DisableRateAdaptive [order 2] : [ActivityLevel < ActivityThreshold]
  DisableRateAdaptive -> RateAdaptiveTransition [order 1] : [(CurrentRate >= DesiredRate) || (ActivityLevel >= ActivityThreshold)]
  DisableRateAdaptive -> DisableRateAdaptive [order 2] : after(1,msec)
  data: ActivityLevel input; ActivityThreshold input; DesiredRate input; ReactionRate input; ReactionRateIncrease input; ReactionRateDecrease input; RecoveryRate input; CurrentRate input

== matlab function AnotherOopsies/RATE_ADAPTIVE/MATLAB Function ==
  data: u input; ActivityLevel output
function ActivityLevel = ActivityScaling(u)
% u = smoothed signal of accel data
% ActivityLevel = scaled number from 0-6
% Activity Threshold = {0,...6}
%                    = {v-low, low, med-low, med, med-high, high, v-high


% u should be between these values
uMin = 10;
uMax = 35;

if (u<uMin)
    u = uMin;
elseif (u>uMax)
    u = uMax;
end


% ActivityLevel = u shifted by -10, then scaled by 6/25
ActivityLevel = 6/25*(u-10);

== stateflow chart AnotherOopsies/COM_IN ==
  state SET_PARAMETERS
    entry:
    %Assign the variable values as received from the DCM
    MODE = typecast(rxdata(3), 'uint8')
    ARP = typecast(rxdata(4:5), 'uint16')
    VRP = typecast(rxdata(6:7), 'uint16')
    ATR_AMPLITUDE = typecast(rxdata(8:11), 'single')
    VENT_AMPLITUDE = typecast(rxdata(12:15), 'single')
    %investigate
    ATR_PULSEWIDTH = typecast(rxdata(16:17), 'uint16')
    VENT_PULSEWIDTH = typecast(rxdata(18:19), 'uint16')
    ATR_CMP_REF_PWM =typecast(rxdata(20), 'uint8')
    VENT_CMP_REF_PWM = typecast(rxdata(21), 'uint8')
    REACTION_TIME=typecast(rxdata(22:23), 'uint16')
    RECOVERY_TIME = typecast(rxdata(24:25), 'uint16')
    PVARP = typecast(rxdata(26), 'uint8')
    FIXED_AV_DELAY = typecast(rxdata(27), 'uint8')
    RESPONSE_FACTOR = typecast(rxdata(28), 'uint8')
    ACTIVITY_THRESHOLD= typecast(rxdata(29), 'uint8')
    LOWER_RATE_LIMIT = typecast(rxdata(30), 'uint8')
    UPPER_RATE_LIMIT =  typecast(rxdata(31), 'uint8')
    MAXIMUM_SENSOR_RATE = typecast(rxdata(32), 'uint8')
  state Initial
    entry:
    %Set Default Input parameters
    MODE = 1;
    ARP = 250;
    VRP = 320;
    ATR_AMPLITUDE = 4.5
    VENT_AMPLITUDE = 4.5
    ATR_PULSEWIDTH = 20
    VENT_PULSEWIDTH = 20
    ATR_CMP_REF_PWM = 90;
    VENT_CMP_REF_PWM = 90;
    REACTION_TIME=10000
    RECOVERY_TIME = 30000
    PVARP = 200
    FIXED_AV_DELAY = 150
    RESPONSE_FACTOR =8
    ACTIVITY_THRESHOLD=1
    LOWER_RATE_LIMIT = 60
    UPPER_RATE_LIMIT =  120
    MAXIMUM_SENSOR_RATE = 120
  state Standby
    %DCM input incoming
  state ECHO_BACK_PARAMETERS
    entry:
    set_params()
  (default) -> Initial
  (junction 11) -> Standby [order 2]
  Initial -> Standby
  (junction 13) -> SET_PARAMETERS [order 1] : [rxdata(2) == 1]
  Standby -> (junction 11) : [status ==0]
  (junction 11) -> (junction 13) [order 1] : [rxdata(1) == 1]
  (junction 13) -> ECHO_BACK_PARAMETERS [order 2] : [rxdata(2) == 2]
  ECHO_BACK_PARAMETERS -> Standby
  data: status input uint8; rxdata input uint8; MODE output uint8; ARP output uint16; VRP output uint16; ATR_AMPLITUDE output single; VENT_AMPLITUDE output single; ATR_PULSEWIDTH output uint16; VENT_PULSEWIDTH output uint16; ATR_CMP_REF_PWM output uint8; VENT_CMP_REF_PWM output uint8; PVARP output uint8; FIXED_AV_DELAY output uint8; UPPER_RATE_LIMIT output uint8; LOWER_RATE_LIMIT output uint8; REACTION_TIME output uint16; RECOVERY_TIME output uint16; RESPONSE_FACTOR output uint8; ACTIVITY_THRESHOLD output uint8; MAXIMUM_SENSOR_RATE output uint8

== matlab function AnotherOopsies/RATE_ADAPTIVE/MATLAB Function1 ==
  data: ActivityLevel input; desiredRate output; ActivityThreshold input; ResponseFactor input
function desiredRate = SetDesiredRate(ActivityLevel, ActivityThreshold, ResponseFactor)

% level = [0,6]
% threshold = [0,6]
% RF = [1,16]

% rate adaptive requirement not met
if (ActivityLevel <= ActivityThreshold) 
    desiredRate = LRL;
    
%rate adapative requirement met (level > threshold), rate adaptive effective
else 
    RFMax = 16;
    thresholdMax = 6;
    scaleCoeff = (MSR - LRL) / (thresholdMax * (RFMax - 1));
    
    desiredRate = (ActivityLevel * ResponseFactor * scaleCoeff) + LRL;
    
end

% ensure desiredRate within boundaries [LRL, MSR]
if desiredRate < LRL
    desiredRate = LRL;

elseif desiredRate > MSR
    desiredRate = MSR;
    
end

== matlab function AnotherOopsies/RATE_ADAPTIVE/MATLAB Function2 ==
  data: MSR input; LRL input; ReactionRate output; ReactionRateIncrease output; ReactionRateDecrease output; ReactionTime input; RecoveryTime input; UpRateSmoothing input; DownRateSmoothing input; CurrentRate input; RecoveryRate output
function [ReactionRate, ReactionRateIncrease, ReactionRateDecrease, RecoveryRate]= SetCurrentSensorControlledRates(MSR, LRL, ReactionTime, RecoveryTime, UpRateSmoothing, DownRateSmoothing, CurrentRate)

secToMsec = 1000;
minToSec = 60;

ReactionRate = (MSR-LRL) / (secToMsec*ReactionTime);
RecoveryRate = (MSR-LRL) / (secToMsec*minToSec*RecoveryTime);


% ensure rate smoothing. 
% ie. rates are within safe values.
maxIncrease = (100 - UpRateSmoothing)*CurrentRate;
maxDecrease = (100 - DownRateSmoothing)*CurrentRate;

% setting safe boundaries
% for ReactionRateIncrease
if (ReactionRate > maxIncrease)
    ReactionRateIncrease = maxIncrease;
else
    ReactionRateIncrease = ReactionRate;
end
% for ReactionRateDecrease
if (ReactionRate > maxDecrease)
    ReactionRateDecrease = maxDecrease;
else
    ReactionRateDecrease = ReactionRate;
end
% for RecoveryRate
if (RecoveryRate > maxDecrease)
    RecoveryRate = maxDecrease;
end
